simulink model "P2_SIL_Model_Diag"  (R2016a)
settings: Solver=ode2  StartTime=0.0  StopTime=Cycle_End  RelTol=1e-3
undefined symbols (not defined in the file): air, APP1_OOR, APP2_OOR, APP_Conversion_IN, APP_Mismatch, bms_inletair_temp, bms_maxchargecurrent, bms_maxdischargecurrent, BMS_Notfallkuehlung, BPP_Flt, cal, clt, ClutchEngag, CrankRequest, dcdc, eng, Engine, EngOverTemp, ENGTRQ_MSMCH_Degraded_CP, ENGTRQ_MSMCH_ErrCritical_CP, ENGTRQ_MSMCH_LimpHome_CP, EngTrqMismatch, env, ess, ESS, ESSOverTemp, fd, FFD, g, gb, Grade, IMG, KeyPos_Flt, KeyPosition, lib_APP_Conversion_IN, lib_ESS_plant_V1_2, lib_OBC_Manager, LossCAN, max_vehicle_rad_air_flow, MCUOverTemp, mot, MotDirMismatch, MotOverTemp, MotTrqMismatch, mph2kph, mph2ms, NeutralGear, obc, OBC_Manager, ParkGear, PRNDL_Flt, ReverseGear, RFD, rho, ShiftLeverPosition, sigbuilder_block, Speed, t_amb, time, tloop ... (+2)
libraries: simulink x104, EC2_libraries x12, Diagnostic x11, lib_CANerror_Detect x3, Utility x1
(part 1 of 11)
settings Model: SimulationMode=accelerator  Creator=Guilin  LastModifiedBy=Guilin
settings OptimizationCC: EfficientMapNaN2IntZero=off
settings HardwareCC: TargetBitPerPointer=64  TargetLongLongMode=on  TargetIntDivRoundTo=Zero  TargetEndianess=LittleEndian  TargetWordSize=64  TargetHWDeviceType=MATLAB Host  ProdEqTarget=off
settings CodeAppCC: MaxIdLength=128
settings GRTTargetCC: GeneratePreprocessorConditionals=Use local settings  CombineOutputUpdateFcns=off  GRTInterface=on

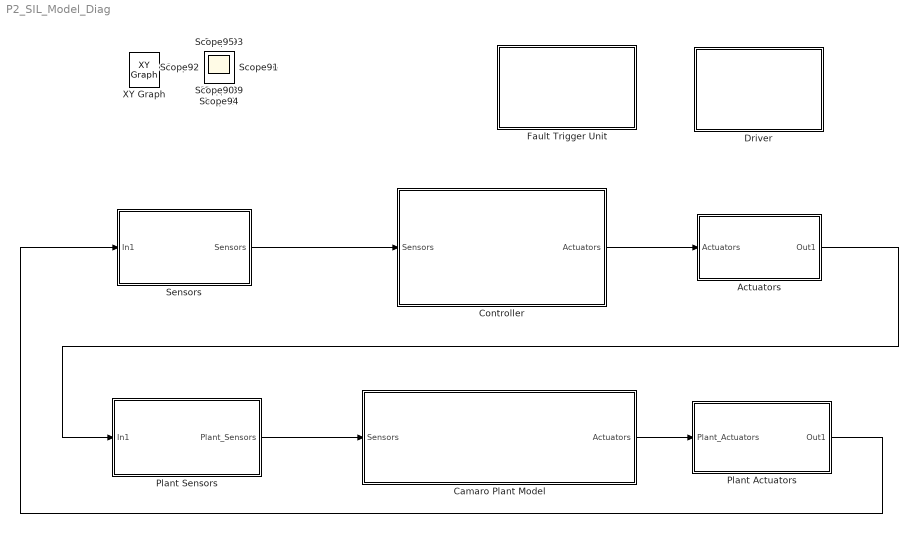
== system P2_SIL_Model_Diag ==
  Actuators : Subsystem
  Camaro Plant Model : Subsystem
      mask Display: image('Images\Vehicle.jpg')
  Controller : Subsystem
      mask Display: image('Images\HCU.jpg')
  Driver : Subsystem
      mask Display: image('Images\Driver.jpg')
  Fault Trigger Unit : Subsystem
  Plant Actuators : Subsystem
  Plant Sensors : Subsystem
  Sensors : Subsystem
  Scope{,1..95} (96 alike) : Scope
  XY Graph : simulink/Sinks/XY Graph  IOType=viewer  xmin=-1  xmax=1  ymin=-1  ymax=1  st=-1
  wires:
  Camaro Plant Model/1(Actuators) -> Plant Actuators/1(Plant_Actuators)
  Plant Sensors/1(Plant_Sensors) -> Camaro Plant Model/1(Sensors)
  Plant Actuators/1(Out1) -> Sensors/1(In1)
  Sensors/1(Sensors) -> Controller/1(Sensors)
  Controller/1(Actuators) -> Actuators/1(Actuators)
  Actuators/1(Out1) -> Plant Sensors/1(In1)

== system P2_SIL_Model_Diag/Actuators ==
  Actuators : Inport
  Analog : Subsystem
  Bus Creator : BusCreator  Inputs=3
  CAN : Subsystem
  Digital : Subsystem
  Ground : Ground
  Out1 : Outport
  wires:
  CAN/1(Out1) -> Bus Creator/1  "to_CAN"
  Analog/1(Out1) -> Bus Creator/2  "to_Analog"
  Digital/1(Out1) -> Bus Creator/3  "to_Digital"
  Actuators/1 -> Digital/1(In1), CAN/1(In1)
  Ground/1 -> Analog/1(In1)
  Bus Creator/1 -> Out1/1

== system P2_SIL_Model_Diag/Camaro Plant Model ==
  Sensors : Inport
  Add : Sum  Inputs=+++
      mask Display:
      | port_label('input',1,'+');
      | port_label('input',2,'+');
      | port_label('input',3,'+');
  Bus Creator : BusCreator  Inputs=2
  Bus Creator1 : BusCreator  Inputs=7
  Bus Selector : BusSelector  OutputSignals=Analog,CAN.to VEH_CAN,CAN.to EBCAN,CAN.to HV_CAN,Digital
  Chassis1 : Subsystem  AncestorBlock=Chassis/Chassis
      mask Display:
      | image('Images/Chassis.jpg');
      | color('red');
      | port_label('input',1,'ShaftIn');
      | port_label('output',1,'SpdOut');
  DC-DC Converter1 : Subsystem  AncestorBlock=DCDC/DC-DC Converter
      mask Display:
      | image('Images\DCDC.png')
      | color('red');
      | port_label('Input',1,'Volt')
      | port_label('Output',1,'Crr')
  Differential : Subsystem  AncestorBlock=Differential/Differential
      mask Display:
      | image('Images/Diff.jpg');
      | color('red');
      | port_label('input',1,'ShaftIn')
      | port_label('input',2,'SpdOut')
      | port_label('output',1,'ShaftOut')
      | port_label('output',2,'SpdIn')
  ESS : Subsystem  AncestorBlock=lib_ESS_plant_V1_2/ESS
      mask Display:
      | image('Images\ESS.jpg')
      | color('red');
      | port_label('Input',1,'Crr');
      | port_label('Output',1,'Volt');
  ICE Simple1 : Subsystem  AncestorBlock=Engine_simple/ICE Simple
      mask Display:
      | image(imread('EngineTopLevel.jpg'),'center')
      | color('red');
      | port_label('input',1,'SpdOut')
      | port_label('output',1,'ShaftOut')
  IMG : Subsystem  AncestorBlock=IMG/IMG
      mask Display:
      | image('Images\Motor.png')
      | color('red');
      | port_label('Input',1,'Volt');
      | port_label('Input',2,'ShaftIn');
      | port_label('Input',3,'SpdOut');
      | port_label('Output',1,'Crr');
      | port_label('Output',2,'ShaftOut');
      | port_label('Output',3,'SpdIn');
  On-Board Charger : Subsystem  AncestorBlock=OBC/On-Board Charger
      mask Display:
      | image('Images\OBC.jpg')
      | color('red');
      | port_label('Input',1,'Volt')
      | port_label('Output',1,'Crr')
  Scopes : Subsystem
      mask Display: image('Images\Scope.jpg')
  Transmission1 : Subsystem  AncestorBlock=Transmission/Transmission
      mask Display:
      | image('Images\Trans.png')
      | color('red');
      | port_label('Input',1,'ShaftIn')
      | port_label('Input',2,'SpdOut')
      | port_label('Output',1,'ShaftOut')
      | port_label('Output',2,'SpdIn')
  Wheels : Subsystem  AncestorBlock=Wheels/Wheels
      mask Display:
      | image('Images/Wheel.jpg');
      | color('red');
      | port_label('input',1,'ShaftIn');
      | port_label('input',2,'SpdOut');
      | port_label('output',1,'ShaftOut');
      | port_label('output',2,'SpdIn');
  Actuators : Outport
  tag scope: Analog=global, Digital=global, HCU_to_EBCAN=global, HCU_to_HV_CAN=global, HCU_to_VEH_CAN=global
  wires:
  Differential/1(fd_shaft_out) -> Wheels/1(whl_shaft_in)
  Wheels/1(whl_shaft_out) -> Chassis1/1(chas_shaft_in)
  Chassis1/1(chas_lin_spd_out) -> Wheels/2(whl_lin_spd_out)
  Differential/2(fd_spd_in) -> Transmission1/2(SpdOut)
  Transmission1/1(ShaftOut) -> Differential/1(fd_shaft_in)
  ESS/1(voltage) -> DC-DC Converter1/1(Volt), IMG/1(voltage), On-Board Charger/1(volt)
  DC-DC Converter1/1(Crr) -> Add/3
  On-Board Charger/1(crr) -> Add/2
  Add/1 -> ESS/1(current)
  Transmission1/2(SpdIn) -> IMG/3(IMG_SpdOut)
  IMG/2(IMG_ShaftOut) -> Transmission1/1(ShaftIn)
  IMG/1(current) -> Add/1
  Bus Creator/1 -> Actuators/1
  Sensors/1 -> Bus Selector/1
  Bus Selector/1 -> [Analog]  "<Analog>"
  Bus Selector/2 -> [HCU_to_VEH_CAN]  "<to VEH_CAN>"
  Bus Selector/3 -> [HCU_to_EBCAN]  "<to EBCAN>"
  Bus Selector/4 -> [HCU_to_HV_CAN]  "<to HV_CAN>"
  Bus Selector/5 -> [Digital]  "<Digital>"
  Wheels/2(whl_spd_in) -> Differential/2(fd_spd_out)
  ICE Simple1/1(eng_shaft_out) -> IMG/2(IMG_ShaftIn)
  IMG/3(IMG_SpdIn) -> ICE Simple1/1(eng_spd_out)
  [ECM_to_HCU] -> Bus Creator1/1
  [TCM_to_HCU] -> Bus Creator1/2
  [BCM_to_HCU] -> Bus Creator1/3
  [BMS_to_HCU] -> Bus Creator1/4
  [MCU_to_HCU] -> Bus Creator1/5
  [APM_to_HCU] -> Bus Creator1/6
  [OBC_to_HCU] -> Bus Creator1/7
  Bus Creator1/1 -> Bus Creator/1  "CAN_to_Actuators"
  [Driver_Request] -> Bus Creator/2  "Driver_Signals"

== system P2_SIL_Model_Diag/Controller ==
  Sensors : Inport
  HSC : Subsystem
  Actuators : Outport
  wires:
  Sensors/1 -> HSC/1(Sensors)
  HSC/1(Actuators) -> Actuators/1

== system P2_SIL_Model_Diag/Driver ==
  Bus Creator : BusCreator  Inputs=6
  Constant : Constant  Commented=on  Value=0
  Driver Control : Subsystem
  Manual Control : Subsystem  Commented=on
  Multiport Switch1 : MultiPortSwitch  Commented=on  DataPortOrder=Zero-based contiguous  Inputs=2
  tag scope: Driver_Request=global
  wires:
  Driver Control/1(Key Position) -> Bus Creator/1  "KeyPos"
  Driver Control/2(APP[%]) -> Bus Creator/2  "drv_APP_req_[%]"
  Driver Control/3(BPP[%]) -> Bus Creator/3  "drv_BPP_req_[%]"
  Driver Control/4(Shift Lever Position) -> Bus Creator/4  "ShiftLvrPos"
  Driver Control/5(EVSE_Pluggin) -> Bus Creator/5  "EVSE_Plugged"
  Constant/1 -> Multiport Switch1/1
  Manual Control/1(Out1) -> Multiport Switch1/3
  Bus Creator/1 -> [Driver_Request]
  Driver Control/6(Veh_Spd) -> Bus Creator/6  "Veh_Spd"

== system P2_SIL_Model_Diag/Fault Trigger Unit ==
  Clock3 : Clock
  Component Diagnostics setting : Subsystem
  Driver Interface Diagnostics setting : Subsystem
  wires:
  Clock3/1 -> Component Diagnostics setting/1(time), Driver Interface Diagnostics setting/1(time)

== system P2_SIL_Model_Diag/Plant Actuators ==
  Plant_Actuators : Inport
  Analog : Subsystem
  Bus Creator : BusCreator  Inputs=3
  Bus Selector : BusSelector  OutputSignals=CAN_to_Actuators,Driver_Signals
  CAN : Subsystem
  Digital : Subsystem  Commented=on
  Out1 : Outport
  wires:
  Bus Creator/1 -> Out1/1  "to_HCU_Sensors"
  Bus Selector/2 -> Analog/1(In1), Digital/1(In1)  "<Driver_Signals>"
  Bus Selector/1 -> CAN/1(In1)  "<CAN_to_Actuators>"
  Plant_Actuators/1 -> Bus Selector/1
  Analog/1(Out1) -> Bus Creator/2  "Analog_to_HCU_Sensors"
  CAN/1(Out1) -> Bus Creator/1  "CAN_to_HCU_Sensors"

== system P2_SIL_Model_Diag/Plant Sensors ==
  In1 : Inport
  Analog : Subsystem
  Bus Creator : BusCreator  Inputs=3
  Bus Selector : BusSelector  OutputSignals=to_CAN,to_Analog,to_Digital
  CAN : Subsystem
  Digital : Subsystem
  Plant_Sensors : Outport
  wires:
  Bus Creator/1 -> Plant_Sensors/1
  Digital/1(Out1) -> Bus Creator/3  "Digital"
  Analog/1(Out1) -> Bus Creator/2  "Analog"
  CAN/1(Out1) -> Bus Creator/1  "CAN"
  In1/1 -> Bus Selector/1
  Bus Selector/1 -> CAN/1(In1)  "<to_CAN>"
  Bus Selector/2 -> Analog/1(In1)  "<to_Analog>"
  Bus Selector/3 -> Digital/1(In1)  "<to_Digital>"

== system P2_SIL_Model_Diag/Sensors ==
  In1 : Inport
  Analog : Subsystem
  Bus Creator : BusCreator  Inputs=3
  Bus Selector : BusSelector  OutputSignals=CAN_to_HCU_Sensors,Analog_to_HCU_Sensors
  CAN : Subsystem
  Digital : Subsystem  Commented=on
  Memory : Memory
  Sensors : Outport
  wires:
  Analog/1(Out1) -> Bus Creator/2  "from_Analog"
  CAN/1(Out1) -> Bus Creator/1  "from_CAN"
  In1/1 -> Bus Selector/1
  Bus Selector/1 -> CAN/1(In1)  "<CAN_to_HCU_Sensors>"
  Bus Selector/2 -> Analog/1(In1)  "<Analog_to_HCU_Sensors>"
  ? -> Digital/1(In1)  "<Digital_to_HCU_Sensors>"
  Bus Creator/1 -> Memory/1
  Memory/1 -> Sensors/1

== system P2_SIL_Model_Diag/Actuators/Analog ==
  In1 : Inport
  Out1 : Outport
  wires:
  In1/1 -> Out1/1

== system P2_SIL_Model_Diag/Actuators/CAN ==
  In1 : Inport
  Bus Creator : BusCreator  Inputs=3
  EBCAN : Subsystem
  HV_CAN : Subsystem
  VEH_CAN : Subsystem
  Out1 : Outport
  wires:
  VEH_CAN/1(Out1) -> Bus Creator/1  "to_VEH_CAN"
  EBCAN/1(Out1) -> Bus Creator/2  "to_EBCAN"
  HV_CAN/1(Out1) -> Bus Creator/3  "to_HV_CAN"
  Bus Creator/1 -> Out1/1  "to_CAN"
  In1/1 -> HV_CAN/1(In1), EBCAN/1(In1), VEH_CAN/1(In1)

== system P2_SIL_Model_Diag/Actuators/Digital ==
  In1 : Inport
  Bus Selector : BusSelector  OutputSignals=BMS_Digital
  Out1 : Outport
  wires:
  In1/1 -> Bus Selector/1
  Bus Selector/1 -> Out1/1  "<BMS_Digital>"

== system P2_SIL_Model_Diag/Camaro Plant Model/Chassis1 ==
  note: Total opposing
      | force (N)
  chas_shaft_in : Inport
  >1 : Saturate  UpperLimit=inf  LowerLimit=0
  Bus Selector : BusSelector  OutputSignals=veh_grade_force_simu,drag force
  Bus Selector1 : BusSelector  OutputSignals=whl_force_out_simu,whl_mass_out_simu
  Clock : Clock
  Driver Interface : Subsystem
  Grade : Lookup  InputValues=time  Table=Grade
  Soft BCM : Subsystem
      mask Display: image('SoftECU.jpg')
  Sum2 : Sum  Inputs=|++  SaturateOnIntegerOverflow=on  InputSameDT=on  OutDataTypeStr=Inherit: Same as first input
  Sum3 : Sum  Inputs=-+  SaturateOnIntegerOverflow=on  InputSameDT=on  OutDataTypeStr=Inherit: Same as first input
  To Workspace1 : ToWorkspace  VariableName=distance_miles_hist  SampleTime=-1
      settings: Decimation=WORKSPACE_DECIMATION
  To Workspace2 : ToWorkspace  VariableName=veh_dist_meter_hist  SampleTime=-1
      settings: Decimation=WORKSPACE_DECIMATION
  To Workspace3 : ToWorkspace  VariableName=veh_spd_mps_hist  SampleTime=-1
      settings: Decimation=WORKSPACE_DECIMATION
  To Workspace7 : ToWorkspace  VariableName=veh_spd_mph_hist  SampleTime=-1
      settings: Decimation=WORKSPACE_DECIMATION
  Velocity1 : Integrator  LimitOutput=on  LowerSaturationLimit=0
  Velocity2 : Integrator  LimitOutput=on  LowerSaturationLimit=0
  m to miles : Gain  Gain=0.00062
  m/s to kph : Gain  Gain=3.6
  ms to mph : Gain  Gain=1/mph2ms
  non-zero division1 : Subsystem
      mask Display: disp('divider \n I1/I2')
  vehicle losses : Subsystem
  vehicle total mass : Constant  Value=veh.init.mass
  chas_lin_spd_out : Outport
  tag scope: BCM_to_HCU=global, chas_plant_force_in=global, chas_plant_force_loss=global, chas_plant_grade=global, chas_plant_lin_accel=global, chas_plant_lin_spd_out=global, chas_plant_mass=global, chas_plant_mass_static=global, veh_dist_miles=global
  wires:
  Grade/1 -> vehicle losses/2(Road grade), [chas_plant_grade]
  Bus Selector/2 -> [chas_plant_force_loss]  "<drag force>"
  Bus Selector/1 -> [chas_plant_force_grade]  "<veh_grade_force_simu>"
  vehicle total mass/1 -> Sum2/1, [chas_plant_mass_static]
  Velocity1/1 -> vehicle losses/1(veh spd simu), m/s to kph/1, Velocity2/1, To Workspace3/1, ms to mph/1, chas_lin_spd_out/1
  non-zero division1/1(Out1) -> Velocity1/1, [chas_plant_lin_accel]
  Sum3/1 -> non-zero division1/1(In1)
  Sum2/1 -> non-zero division1/2(In2), [chas_plant_mass]
  >1/1 -> Sum2/2
  Bus Selector1/2 -> >1/1  "<whl_mass_out_simu>"
  Bus Selector1/1 -> Sum3/2, [chas_plant_force_in]  "<whl_force_out_simu>"
  chas_shaft_in/1 -> Bus Selector1/1
  vehicle losses/1(info) -> Bus Selector/1
  vehicle losses/2(veh_force_loss_simu) -> Sum3/1
  Soft BCM/1(Out1) -> [BCM_to_HCU]
  m/s to kph/1 -> [chas_plant_lin_spd_out]
  ms to mph/1 -> To Workspace7/1
  Clock/1 -> Grade/1
  Velocity2/1 -> To Workspace2/1, m to miles/1
  m to miles/1 -> [veh_dist_miles], To Workspace1/1

== system P2_SIL_Model_Diag/Camaro Plant Model/DC-DC Converter1 ==
  Volt : Inport
  Eff : Gain  Gain=1/dcdc.init.eff
  Electrical Accessory Load : Constant  Value=dcdc.init.constant_pwr
  Subsystem2 : Subsystem
      mask Display: disp('divider')
  Crr : Outport
  wires:
  Eff/1 -> Subsystem2/1(In1)
  Subsystem2/1(Out1) -> Crr/1
  Electrical Accessory Load/1 -> Eff/1
  Volt/1 -> Subsystem2/2(In2)

== system P2_SIL_Model_Diag/Camaro Plant Model/Differential ==
  fd_shaft_in : Inport
  fd_spd_out : Inport  Port=2
  Bus Creator : BusCreator  Inputs=2
  Bus Selector : BusSelector  OutputSignals=gb_trq_out,gb_inertia_out
  Inertia calculation : Subsystem
  Speed calculation : Subsystem
  Torque calculation : Subsystem
  fd_shaft_out : Outport
  fd_spd_in : Outport  Port=2
  wires:
  Torque calculation/1(trq out) -> Bus Creator/1  "fd_trq_out_simu"
  fd_spd_out/1 -> Speed calculation/1(spd out)
  Speed calculation/1(spd in) -> Torque calculation/1(spd in), fd_spd_in/1
  Inertia calculation/1(inertia out) -> Bus Creator/2  "fd_inertia_out_simu"
  Bus Selector/1 -> Torque calculation/2(trq in)  "<gb_trq_out>"
  Bus Selector/2 -> Inertia calculation/1(inertia in)  "<gb_inertia_out>"
  fd_shaft_in/1 -> Bus Selector/1
  Bus Creator/1 -> fd_shaft_out/1

== system P2_SIL_Model_Diag/Camaro Plant Model/ESS ==
  note: BMS_to_Actuators
  current : Inport
  ESS : Subsystem
      mask Display:
      | image('Images\ESS.jpg')
      | color('red');
      | port_label('Input',2,'Crr');
      | port_label('Output',2,'Volt');
  Inputs : Subsystem  AncestorBlock=lib_DCDC/DC-DC Converter/Inputs
  Outputs : Subsystem
  Soft BMS : Subsystem  RequirementInfo={} %GIDa_a1686922_eaef_470c_99b9_57900de5863a
      mask Display: image('softECU.jpg')
  voltage : Outport
  wires:
  current/1 -> ESS/2("Crr ")
  Soft BMS/2(Output2) -> ESS/1("In ")
  ESS/1(out) -> Soft BMS/2(Input2)  "Sensors_to_BMS"
  ESS/2(Voltage) -> voltage/1
  Soft BMS/1(CAN) -> Outputs/1(Outputs)
  Inputs/1(Inputs) -> Soft BMS/1(Input1)

== system P2_SIL_Model_Diag/Camaro Plant Model/ICE Simple1 ==
  eng_spd_out : Inport
  Engine Plant Modified : Subsystem
      mask Display:
      | image(imread('EngineTopLevel.jpg'),'center')
      | color('red');
      | port_label('input',2,'SpdOut')
      | port_label('output',2,'ShaftOut')
  Inputs : Subsystem
  Soft ECM : Subsystem
      mask Display: image('SoftECU.jpg')
  eng_shaft_out : Outport
  tag scope: ECM_to_HCU=global
  wires:
  Engine Plant Modified/2(eng_shaft_out) -> eng_shaft_out/1
  eng_spd_out/1 -> Engine Plant Modified/2(eng_spd_out)
  Soft ECM/2(Out1) -> Engine Plant Modified/1("In ")  "ECM_to_Actuators"
  Inputs/1(Inputs) -> Soft ECM/1(In)
  Soft ECM/1(Out) -> [ECM_to_HCU]
  Engine Plant Modified/1(Out) -> Soft ECM/2(In1)

== system P2_SIL_Model_Diag/Camaro Plant Model/IMG ==
  voltage : Inport
  IMG_ShaftIn : Inport  Port=2
  IMG_SpdOut : Inport  Port=3
  IMG Plant : Subsystem
      mask Display:
      | image('Images\Motor.png')
      | color('red');
      | port_label('Input',2,'Volt');
      | port_label('Input',3,'ShaftIn');
      | port_label('Input',4,'SpdOut');
      | port_label('Output',2,'Crr');
      | port_label('Output',3,'ShaftOut');
      | port_label('Output',4,'SpdIn');
  Soft MCU : Subsystem
      mask Display: image('softECU.jpg')
  current : Outport
  IMG_ShaftOut : Outport  Port=2
  IMG_SpdIn : Outport  Port=3
  tag scope: MCU_to_HCU=global
  wires:
  IMG Plant/1(Out1) -> Soft MCU/2(In1)  "Sensors_to_MCU"
  Soft MCU/2(Out1) -> IMG Plant/1("In1 ")  "MCU_to_Actuators"
  Soft MCU/1(Out) -> [MCU_to_HCU]
  [HCU_to_HV_CAN] -> Soft MCU/1(In)
  IMG_SpdOut/1 -> IMG Plant/4(SpdOut)
  IMG Plant/4(SpdIn) -> IMG_SpdIn/1
  IMG Plant/2(current) -> current/1
  voltage/1 -> IMG Plant/2(voltage)
  IMG Plant/3(MotShaftOut) -> IMG_ShaftOut/1
  IMG_ShaftIn/1 -> IMG Plant/3(MotShaftIn)

== system P2_SIL_Model_Diag/Camaro Plant Model/On-Board Charger ==
  volt : Inport
  HCU to OBC : Subsystem
  OBC to HCU : Subsystem
  On Board Charger : Subsystem
      mask Display:
      | image('Images\OBC.jpg')
      | color('red');
      | port_label('Input',1,'Volt')
      | port_label('Output',1,'Crr')
  Soft_OBC : Subsystem
      mask Display: image('softECU.jpg')
  crr : Outport
  wires:
  volt/1 -> On Board Charger/2(volt)
  On Board Charger/2(crr) -> crr/1
  HCU to OBC/1(Inputs) -> Soft_OBC/1(Inputs)
  Soft_OBC/1(Outputs) -> OBC to HCU/1(Outputs)
  On Board Charger/1(Out1) -> Soft_OBC/2(Inputs1)  "Sensors_to_OBC"
  Soft_OBC/2(Outputs1) -> On Board Charger/1("In1 ")  "OBC_to_Actuators"

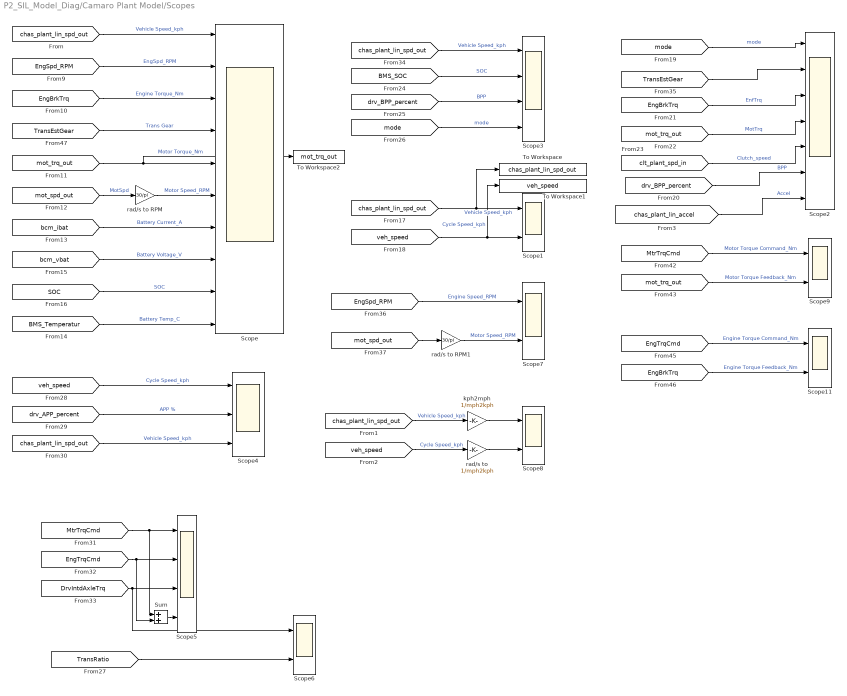
== system P2_SIL_Model_Diag/Camaro Plant Model/Scopes ==
  Scope : Scope  NumInputPorts=10
  Scope{1,6..9,11} (6 alike) : Scope  NumInputPorts=2
  Scope2 : Scope  NumInputPorts=7
  Scope3 : Scope  NumInputPorts=4
  Scope4 : Scope  NumInputPorts=3
  Scope5 : Scope  NumInputPorts=4
  Sum : Sum
  To Workspace : ToWorkspace  VariableName=chas_plant_lin_spd_out  SaveFormat=Timeseries  SampleTime=-1
  To Workspace1 : ToWorkspace  VariableName=veh_speed  SaveFormat=Timeseries  SampleTime=-1
  To Workspace2 : ToWorkspace  VariableName=mot_trq_out  SaveFormat=Timeseries  SampleTime=-1
  kph2mph : Gain  Gain=1/mph2kph
  "rad/s to " : Gain  Gain=1/mph2kph
  rad/s to RPM : Gain  Gain=30/pi
  rad/s to RPM1 : Gain  Gain=30/pi
  wires:
  [chas_plant_lin_spd_out] -> Scope/1  "Vehicle Speed_kph"
  [EngSpd_RPM] -> Scope/2  "EngSpd_RPM"
  [EngBrkTrq] -> Scope/3  "Engine Torque_Nm"
  [mot_spd_out] -> rad/s to RPM/1  "MotSpd"
  [BMS_Temperatur] -> Scope/10  "Battery Temp_C"
  rad/s to RPM/1 -> Scope/6  "Motor Speed_RPM"
  [mot_trq_out] -> To Workspace2/1, Scope/5  "Motor Torque_Nm"
  [bcm_vbat] -> Scope/8  "Battery Voltage_V"
  [SOC] -> Scope/9  "SOC"
  [TransEstGear] -> Scope/4  "Trans Gear"
  [bcm_ibat] -> Scope/7  "Battery Current_A"
  [chas_plant_lin_spd_out] -> Scope3/1  "Vehicle Speed_kph"
  [BMS_SOC] -> Scope3/2  "SOC"
  [drv_BPP_percent] -> Scope3/3  "BPP"
  [mode] -> Scope3/4  "mode"
  [chas_plant_lin_spd_out] -> To Workspace/1, Scope1/1  "Vehicle Speed_kph"
  [veh_speed] -> To Workspace1/1, Scope1/2  "Cycle Speed_kph"
  [mode] -> Scope2/1  "mode"
  [EngBrkTrq] -> Scope2/3  "EnfTrq"
  [mot_trq_out] -> Scope2/4  "MotTrq"
  [clt_plant_spd_in] -> Scope2/5  "Clutch_speed"
  [EngSpd_RPM] -> Scope7/1  "Engine Speed_RPM"
  [mot_spd_out] -> rad/s to RPM1/1
  rad/s to RPM1/1 -> Scope7/2  "Motor Speed_RPM"
  [veh_speed] -> Scope4/1  "Cycle Speed_kph"
  [drv_APP_percent] -> Scope4/2  "APP %"
  [chas_plant_lin_spd_out] -> Scope4/3  "Vehicle Speed_kph"
  [MtrTrqCmd] -> Sum/1, Scope5/1
  [EngTrqCmd] -> Sum/2, Scope5/2
  [DrvIntdAxleTrq] -> Scope6/1, Scope5/3
  Sum/1 -> Scope5/4
  [TransRatio] -> Scope6/2
  [MtrTrqCmd] -> Scope9/1  "Motor Torque Command_Nm"
  [mot_trq_out] -> Scope9/2  "Motor Torque Feedback_Nm"
  [EngTrqCmd] -> Scope11/1  "Engine Torque Command_Nm"
  [EngBrkTrq] -> Scope11/2  "Engine Torque Feedback_Nm"
  [chas_plant_lin_spd_out] -> kph2mph/1  "Vehicle Speed_kph"
  [veh_speed] -> "rad/s to "/1  "Cycle Speed_kph"
  kph2mph/1 -> Scope8/1
  "rad/s to "/1 -> Scope8/2
  [TransEstGear] -> Scope2/2
  [drv_BPP_percent] -> Scope2/6  "BPP"
  [chas_plant_lin_accel] -> Scope2/7  "Accel"

== system P2_SIL_Model_Diag/Camaro Plant Model/Transmission1 ==
  ShaftIn : Inport
  SpdOut : Inport  Port=2
  Inputs : Subsystem  AncestorBlock=lib_DCDC/DC-DC Converter/Inputs
  Outputs : Subsystem  AncestorBlock=lib_DCDC/DC-DC Converter/Outputs
  Soft TCM : Subsystem
      mask Display: image('softECU.jpg')
  Transmission Plant : Subsystem
      mask Display:
      | image('Images\Trans.png')
      | color('red');
      | port_label('Input',2,'ShaftIn')
      | port_label('Input',3,'SpdOut')
      | port_label('Output',2,'ShaftOut')
      | port_label('Output',3,'SpdIn')
  ShaftOut : Outport
  SpdIn : Outport  Port=2
  wires:
  Transmission Plant/3(TorqConvSpdIn) -> SpdIn/1
  Transmission Plant/2(GearboxShaftOut) -> ShaftOut/1
  SpdOut/1 -> Transmission Plant/3(GearboxSpdOut)
  ShaftIn/1 -> Transmission Plant/2(TorqConvShaftIn)
  Soft TCM/1(Out) -> Outputs/1(Outputs)
  Inputs/1(Inputs) -> Soft TCM/1(In)
  Transmission Plant/1(Out1) -> Soft TCM/2(In1)  "Sensors_to_TCM"
  Soft TCM/2(Out1) -> Transmission Plant/1("In1 ")  "TCM_to_Actuators"

== system P2_SIL_Model_Diag/Camaro Plant Model/Wheels ==
  whl_shaft_in : Inport
  whl_lin_spd_out : Inport  Port=2
  "1\\radius " : Gain  Gain=1/whl.plant.init.radius  SaturateOnIntegerOverflow=on  OutDataTypeStr=Inherit: Same as input  ParamDataTypeStr=Inherit: Same as input
  Bus Creator : BusCreator  Inputs=2
  Bus Selector : BusSelector  OutputSignals=drv_BPP_req_[%]
  Bus Selector1 : BusSelector  OutputSignals=fd_trq_out_simu,fd_inertia_out_simu
  Clock : Clock
  Force calculation : Subsystem
  Grade : Lookup  InputValues=time  Table=Grade
  Mass calculation : Subsystem
  Speed calculation : Subsystem
  whl_shaft_out : Outport
  whl_spd_in : Outport  Port=2
  wires:
  Bus Selector/1 -> Force calculation/2(BPP[%])  "<drv_BPP_req_[%]>"
  [Driver_Request] -> Bus Selector/1
  "1\\radius "/1 -> Speed calculation/1(chas_spd)
  Force calculation/1(force) -> Bus Creator/1  "whl_force_out_simu"
  Speed calculation/1(spd in) -> Force calculation/1(spd in), whl_spd_in/1
  Mass calculation/1(Mass) -> Bus Creator/2  "whl_mass_out_simu"
  Bus Selector1/1 -> Force calculation/5(trq_in)  "<fd_trq_out_simu>"
  Bus Selector1/2 -> Mass calculation/1(inertia in)  "<fd_inertia_out_simu>"
  whl_lin_spd_out/1 -> "1\\radius "/1, Force calculation/3(whl_spd)
  whl_shaft_in/1 -> Bus Selector1/1
  Bus Creator/1 -> whl_shaft_out/1
  Grade/1 -> Force calculation/4(grade)
  Clock/1 -> Grade/1

== system P2_SIL_Model_Diag/Controller/HSC ==
  Sensors : Inport
  Camaro Fault Detection : Subsystem  AncestorBlock=Diagnostic/Camaro Diagnostic
  Driver_Requests : Subsystem  RequirementInfo="{'other' 'HCU_Requirements.xlsx' '@Simulink_requirement_item_5' 'true' 'Determines the  driver''s intention i.e. status of the vehicle start, HCU on/off status and the Driver Intend Axle Torque from the sensor inputs.' '' } %GIDa_43b9b296_ab65_412c_9ca4_dcb3f85d1554"
  Ground : Ground
  Powertrain Manager : Subsystem
  Actuators : Outport
  wires:
  Sensors/1 -> Driver_Requests/1(Sensors), Camaro Fault Detection/1(Sensors), Powertrain Manager/1(Sensors)
  Powertrain Manager/1(Out1) -> Actuators/1
  Ground/1 -> Driver_Requests/2(Diagnostics)
  Driver_Requests/1(DriverRequests) -> Powertrain Manager/2(Driver Request)
  Camaro Fault Detection/1(Out2) -> Powertrain Manager/3(Fault Detection)

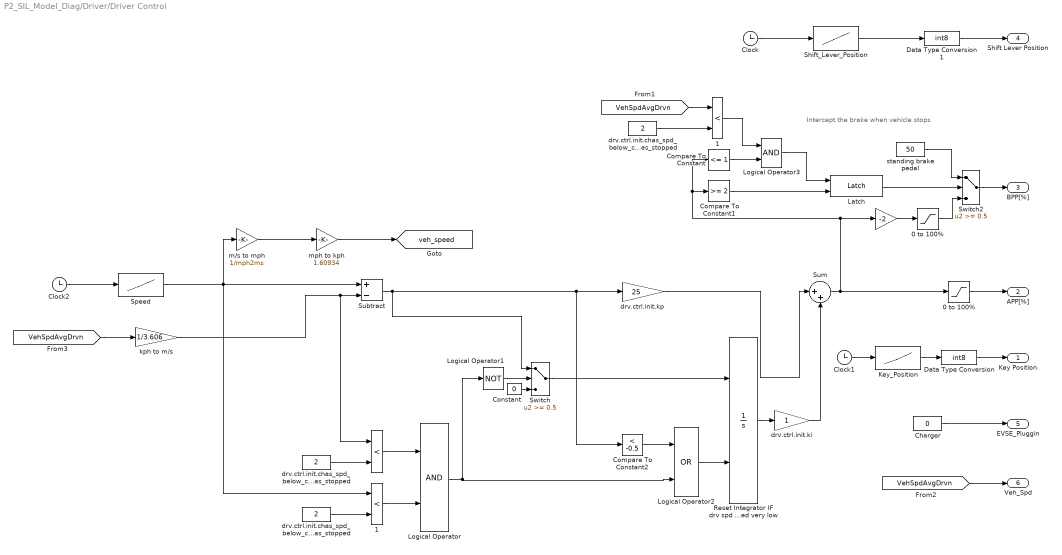
== system P2_SIL_Model_Diag/Driver/Driver Control ==
  note: Intercept the brake when vehicle stops
  " " : Gain  Gain=-2
  "    " : RelationalOperator  Operator=<  InputSameDT=on
  "    1" : RelationalOperator  Operator=<  InputSameDT=on
  "  1" : RelationalOperator  Operator=<  InputSameDT=on
  0 to 100% : Saturate  UpperLimit=100  LowerLimit=0
  "0 to 100% " : Saturate  UpperLimit=100  LowerLimit=0
  Charger : Constant  Value=0
  Clock : Clock
  Clock1 : Clock
  Clock2 : Clock
  Compare To Constant : simulink/Logic and Bit Operations/Compare To Constant  relop=<=  const=1  OutDataTypeStr=boolean
  Compare To Constant1 : simulink/Logic and Bit Operations/Compare To Constant  relop=>=  const=2  OutDataTypeStr=boolean
  Compare To Constant2 : simulink/Logic and Bit Operations/Compare To Constant  relop=<  const=-0.5  OutDataTypeStr=boolean
  Constant : Constant  Value=0
  Data Type Conversion : DataTypeConversion  OutDataTypeStr=int8
  Data Type Conversion1 : DataTypeConversion  OutDataTypeStr=int8
  Key_Position : Lookup  InputValues=time  Table=KeyPosition
  Latch : Utility/Latch
  Logical Operator : Logic  AllPortsSameDT=off  OutDataTypeStr=boolean
  Logical Operator1 : Logic  Operator=NOT  AllPortsSameDT=off  OutDataTypeStr=boolean
  Logical Operator2 : Logic  Operator=OR  AllPortsSameDT=off  OutDataTypeStr=boolean
  Logical Operator3 : Logic  AllPortsSameDT=off  OutDataTypeStr=boolean
  Reset Integrator IF drv spd dmd very low AND AND current vehicle speed very low : Integrator  ExternalReset=either
  Shift_Lever_Position : Lookup  InputValues=time  Table=ShiftLeverPosition
  Speed : Lookup  InputValues=time  Table=Speed
  Subtract : Sum  Inputs=+-
  Sum : Sum  Inputs=|++  SaturateOnIntegerOverflow=on  InputSameDT=on  OutDataTypeStr=Inherit: Same as first input
  Switch : Switch  Threshold=0.5
  Switch2 : Switch  Threshold=0.5
  "drv.ctrl.init.chas_spd_below_chas_stopped " : Constant  Value=2
  "drv.ctrl.init.chas_spd_below_chas_stopped " : Constant  Value=2
  "drv.ctrl.init.chas_spd_below_chas_stopped " : Constant  Value=2
  drv.ctrl.init.ki : Gain  SaturateOnIntegerOverflow=on  OutDataTypeStr=Inherit: Same as input  ParamDataTypeStr=Inherit: Same as input
  drv.ctrl.init.kp : Gain  Gain=25  SaturateOnIntegerOverflow=on  OutDataTypeStr=Inherit: Same as input  ParamDataTypeStr=Inherit: Same as input
  kph to m/s : Gain  Gain=1/3.606  SaturateOnIntegerOverflow=on  OutDataTypeStr=Inherit: Same as input  ParamDataTypeStr=Inherit: Same as input
  m/s to mph : Gain  Gain=1/mph2ms
  mph to kph : Gain  Gain=1.60934
  standing brake pedal : Constant  Value=50
  Key Position : Outport
  APP[%] : Outport  Port=2
  BPP[%] : Outport  Port=3
  Shift Lever Position : Outport  Port=4
  EVSE_Pluggin : Outport  Port=5
  Veh_Spd : Outport  Port=6
  tag scope: veh_speed=global
  wires:
  drv.ctrl.init.kp/1 -> Sum/1
  "    "/1 -> Logical Operator/1
  Speed/1 -> Subtract/1, m/s to mph/1, "  1"/1
  Constant/1 -> Switch/3
  Reset Integrator IF drv spd dmd very low AND AND current vehicle speed very low/1 -> drv.ctrl.init.ki/1
  kph to m/s/1 -> Subtract/2, "    "/1
  Logical Operator1/1 -> Switch/2
  "drv.ctrl.init.chas_spd_below_chas_stopped "/1 -> "    "/2
  Switch/1 -> Reset Integrator IF drv spd dmd very low AND AND current vehicle speed very low/1
  Logical Operator2/1 -> Reset Integrator IF drv spd dmd very low AND AND current vehicle speed very low/2
  "drv.ctrl.init.chas_spd_below_chas_stopped "/1 -> "  1"/2
  drv.ctrl.init.ki/1 -> Sum/2
  "  1"/1 -> Logical Operator/2
  Logical Operator/1 -> Logical Operator2/2, Logical Operator1/1
  "0 to 100% "/1 -> Switch2/3
  " "/1 -> "0 to 100% "/1
  [VehSpdAvgDrvn] -> kph to m/s/1
  standing brake pedal/1 -> Switch2/1
  Switch2/1 -> BPP[%]/1
  [VehSpdAvgDrvn] -> "    1"/1
  "drv.ctrl.init.chas_spd_below_chas_stopped "/1 -> "    1"/2
  "    1"/1 -> Logical Operator3/1
  Sum/1 -> Compare To Constant1/1, Compare To Constant/1, " "/1, 0 to 100%/1
  Logical Operator3/1 -> Latch/1
  Compare To Constant/1 -> Logical Operator3/2
  Compare To Constant1/1 -> Latch/2
  Latch/1 -> Switch2/2
  Shift_Lever_Position/1 -> Data Type Conversion1/1
  Data Type Conversion/1 -> Key Position/1
  Data Type Conversion1/1 -> Shift Lever Position/1
  Charger/1 -> EVSE_Pluggin/1
  Subtract/1 -> Compare To Constant2/1, drv.ctrl.init.kp/1, Switch/1
  Compare To Constant2/1 -> Logical Operator2/1
  Clock/1 -> Shift_Lever_Position/1
  Clock1/1 -> Key_Position/1
  Key_Position/1 -> Data Type Conversion/1
  Clock2/1 -> Speed/1
  m/s to mph/1 -> mph to kph/1
  mph to kph/1 -> [veh_speed]
  0 to 100%/1 -> APP[%]/1
  [VehSpdAvgDrvn] -> Veh_Spd/1

== system P2_SIL_Model_Diag/Driver/Manual Control ==
  note: Manipulate these values
      | to drive vehicle
  APP[%] : Constant
  BPP[%] : Constant  Value=-1
  Bus Creator1 : BusCreator  Inputs=5
  KeyPosition : Constant  Value=3
  PRNDL : Constant  Value=4
  ReferenceVel1 : Constant  Value=0
  Saturation : Saturate  UpperLimit=100  LowerLimit=0
  Saturation1 : Saturate  UpperLimit=0  LowerLimit=-100
  Saturation2 : Saturate  UpperLimit=3  LowerLimit=0
  Saturation3 : Saturate  UpperLimit=4  LowerLimit=0
  Slider Gain : simulink/Math Operations/Slider Gain  low=0  gain=0  high=100
  Slider Gain1 : simulink/Math Operations/Slider Gain  low=0  gain=0  high=100
  Out1 : Outport
  wires:
  Saturation2/1 -> Bus Creator1/3  "Key_Pos_[0_3]"
  Saturation1/1 -> Bus Creator1/2  "BPP(%)"
  Saturation/1 -> Bus Creator1/1  "APP (%)"
  KeyPosition/1 -> Saturation2/1
  Bus Creator1/1 -> Out1/1  "DriverOut"
  BPP[%]/1 -> Slider Gain1/1
  APP[%]/1 -> Slider Gain/1
  ReferenceVel1/1 -> Bus Creator1/5  "refVel [m/s]"
  PRNDL/1 -> Saturation3/1
  Saturation3/1 -> Bus Creator1/4  "PRNDL"
  Slider Gain/1 -> Saturation/1
  Slider Gain1/1 -> Saturation1/1

== system P2_SIL_Model_Diag/Fault Trigger Unit/Component Diagnostics setting ==
  time : Inport
  ClutchEngag : Lookup  Commented=on  InputValues=time  Table=ClutchEngag  LookUpMeth=Interpolation-Use End Values  OutDataTypeStr=int8
  ESSOverTemp : Lookup  Commented=on  InputValues=time  Table=ESSOverTemp  LookUpMeth=Interpolation-Use End Values  OutDataTypeStr=int8
  EngOverTemp : Lookup  Commented=on  InputValues=time  Table=EngOverTemp  LookUpMeth=Interpolation-Use End Values  OutDataTypeStr=int8
  EngTrqMismatch : Lookup  Commented=on  InputValues=time  Table=EngTrqMismatch  LookUpMeth=Interpolation-Use End Values  OutDataTypeStr=int8
  Goto1 : Goto  Commented=on  GotoTag=MotTrqMismatch  TagVisibility=global
  Goto2 : Goto  Commented=on  GotoTag=LossCAN_ON  TagVisibility=global
  Goto3 : Goto  Commented=on  GotoTag=EngTrqMismatch  TagVisibility=global
  Goto4 : Goto  Commented=on  GotoTag=MotOverTemp  TagVisibility=global
  Goto5 : Goto  Commented=on  GotoTag=MCUOverTemp  TagVisibility=global
  Goto6 : Goto  Commented=on  GotoTag=MotDirMismatch  TagVisibility=global
  Goto7 : Goto  Commented=on  GotoTag=EngOverTemp  TagVisibility=global
  Goto8 : Goto  Commented=on  GotoTag=ESSOverTemp  TagVisibility=global
  Goto9 : Goto  Commented=on  GotoTag=ClutchEngagFlt  TagVisibility=global
  LossCAN : Lookup  Commented=on  InputValues=time  Table=LossCAN  LookUpMeth=Interpolation-Use End Values  OutDataTypeStr=int8
  MCUOverTemp : Lookup  Commented=on  InputValues=time  Table=MCUOverTemp  LookUpMeth=Interpolation-Use End Values  OutDataTypeStr=int8
  Mismch type : Subsystem  Commented=on
  Mismch type1 : Subsystem  Commented=on
  MotDirMismatch : Lookup  Commented=on  InputValues=time  Table=MotDirMismatch  LookUpMeth=Interpolation-Use End Values  OutDataTypeStr=int8
  MotOverTemp : Lookup  Commented=on  InputValues=time  Table=MotOverTemp  LookUpMeth=Interpolation-Use End Values  OutDataTypeStr=int8
  MotTrqMismatch : Lookup  Commented=on  InputValues=time  Table=MotTrqMismatch  LookUpMeth=Interpolation-Use End Values  OutDataTypeStr=int8
  Override  ClutchEngag : Subsystem  Commented=on
  Override  ESSOverTemp : Subsystem  Commented=on
  Override  EngOverTemp : Subsystem  Commented=on
  Override  EngTrqMismatch : Subsystem  Commented=on
  Override  LossCAN : Subsystem  Commented=on
  Override  MCUOverTemp : Subsystem  Commented=on
  Override  MotDirMismatch : Subsystem  Commented=on
  Override  MotOverTemp : Subsystem  Commented=on
  Override  MotTrqMismatch : Subsystem  Commented=on
  wires:
  MotOverTemp/1 -> Override  MotOverTemp/1(In1)
  LossCAN/1 -> Override  LossCAN/1(In1)
  time/1 -> LossCAN/1, MotTrqMismatch/1, EngTrqMismatch/1, MotOverTemp/1, MCUOverTemp/1, EngOverTemp/1, ClutchEngag/1, ESSOverTemp/1, MotDirMismatch/1
  Override  LossCAN/1(Out1) -> Goto2/1
  Override  MCUOverTemp/1(Out1) -> Goto5/1
  Override  EngTrqMismatch/1(Out1) -> Goto3/1
  Override  MotDirMismatch/1(Out1) -> Goto6/1
  MotDirMismatch/1 -> Override  MotDirMismatch/1(In1)
  Override  MotTrqMismatch/1(Out1) -> Goto1/1
  MotTrqMismatch/1 -> Mismch type1/1(In1)
  EngTrqMismatch/1 -> Mismch type/1(In1)
  Override  MotOverTemp/1(Out1) -> Goto4/1
  MCUOverTemp/1 -> Override  MCUOverTemp/1(In1)
  Override  EngOverTemp/1(Out1) -> Goto7/1
  EngOverTemp/1 -> Override  EngOverTemp/1(In1)
  Override  ESSOverTemp/1(Out1) -> Goto8/1
  ESSOverTemp/1 -> Override  ESSOverTemp/1(In1)
  Override  ClutchEngag/1(Out1) -> Goto9/1
  ClutchEngag/1 -> Override  ClutchEngag/1(In1)
  Mismch type/1(Out1) -> Override  EngTrqMismatch/1(In1)
  Mismch type1/1(Out1) -> Override  MotTrqMismatch/1(In1)

== system P2_SIL_Model_Diag/Fault Trigger Unit/Driver Interface Diagnostics setting ==
  time : Inport
  APP1_OOR : Lookup  Commented=on  InputValues=time  Table=APP1_OOR  LookUpMeth=Interpolation-Use End Values  OutDataTypeStr=int8
  APP2_OOR : Lookup  Commented=on  InputValues=time  Table=APP2_OOR  LookUpMeth=Interpolation-Use End Values  OutDataTypeStr=int8
  APP_Mismatch : Lookup  Commented=on  InputValues=time  Table=APP_Mismatch  LookUpMeth=Interpolation-Use End Values  OutDataTypeStr=int8
  BPP_Flt : Lookup  Commented=on  InputValues=time  Table=BPP_Flt  LookUpMeth=Interpolation-Use End Values  OutDataTypeStr=int8
  Goto1 : Goto  Commented=on  GotoTag=APP1_OOR_ON  TagVisibility=global
  Goto3 : Goto  Commented=on  GotoTag=BPP_Flt  TagVisibility=global
  Goto4 : Goto  Commented=on  GotoTag=KeyPos_Flt_ON  TagVisibility=global
  Goto5 : Goto  Commented=on  GotoTag=PRNDL_Flt_ON  TagVisibility=global
  Goto6 : Goto  Commented=on  GotoTag=APP2_OOR_ON  TagVisibility=global
  Goto7 : Goto  Commented=on  GotoTag=Mismatch_APP_ON  TagVisibility=global
  KeyPos_Flt : Lookup  Commented=on  InputValues=time  Table=KeyPos_Flt  LookUpMeth=Interpolation-Use End Values  OutDataTypeStr=int8
  Override  APP1_OOR : Subsystem  Commented=on
  Override  APP2_OOR : Subsystem  Commented=on
  Override  APP_Mismatch : Subsystem  Commented=on
  Override  BPP_Flt : Subsystem  Commented=on
  Override  KeyPos_Flt : Subsystem  Commented=on
  Override  PRNDL_Flt : Subsystem  Commented=on
  PRNDL_Flt : Lookup  Commented=on  InputValues=time  Table=PRNDL_Flt  LookUpMeth=Interpolation-Use End Values  OutDataTypeStr=int8
  To Workspace : ToWorkspace  Commented=on  VariableName=APP_Mismatch  SaveFormat=Timeseries  SampleTime=-1
  wires:
  PRNDL_Flt/1 -> Override  PRNDL_Flt/1(In1)
  Override  KeyPos_Flt/1(Out1) -> Goto4/1
  BPP_Flt/1 -> Override  BPP_Flt/1(In1)
  APP1_OOR/1 -> Override  APP1_OOR/1(In1)
  Override  APP1_OOR/1(Out1) -> Goto1/1
  APP2_OOR/1 -> Override  APP2_OOR/1(In1)
  Override  APP2_OOR/1(Out1) -> Goto6/1
  Override  BPP_Flt/1(Out1) -> Goto3/1
  Override  PRNDL_Flt/1(Out1) -> Goto5/1
  time/1 -> APP_Mismatch/1, APP2_OOR/1, PRNDL_Flt/1, KeyPos_Flt/1, BPP_Flt/1, APP1_OOR/1
  KeyPos_Flt/1 -> Override  KeyPos_Flt/1(In1)
  Override  APP_Mismatch/1(Out1) -> To Workspace/1, Goto7/1
  APP_Mismatch/1 -> Override  APP_Mismatch/1(In1)

== system P2_SIL_Model_Diag/Plant Actuators/Analog ==
  In1 : Inport
  APP_Fault_Insertion : Subsystem
  APP_to_APP1_Recast : Subsystem
  APP_to_APP2_Recast : Subsystem
  Bus Creator : BusCreator  Inputs=5
  Bus Creator1 : BusCreator  Inputs=2
  Bus Selector : BusSelector  OutputSignals=drv_APP_req_[%],ShiftLvrPos,KeyPos,drv_BPP_req_[%]
  Switch : Switch  Criteria=u2 > Threshold
  Out1 : Outport
  wires:
  Bus Creator/1 -> Out1/1  "Analog"
  Bus Selector/4 -> Bus Creator/5  "<drv_BPP_req_[%]>"
  Bus Selector/3 -> Bus Creator/4  "<KeyPos>"
  Bus Selector/2 -> Bus Creator/3  "<ShiftLvrPos>"
  In1/1 -> Bus Selector/1
  Bus Selector/1 -> Bus Creator/1, APP_Fault_Insertion/1(AccPos)  "<drv_APP_req_[%]>"
  APP_Fault_Insertion/1(APP1) -> APP_to_APP1_Recast/1(APP1_IN)
  APP_Fault_Insertion/2(APP2) -> APP_to_APP2_Recast/1(APP2_IN)
  APP_to_APP1_Recast/1(APP1Recast) -> Bus Creator1/1  "Driver_APP1"
  APP_to_APP2_Recast/1(APP2Recast) -> Bus Creator1/2  "Driver_APP2"
  Bus Creator1/1 -> Bus Creator/2  "APP_Out"

== system P2_SIL_Model_Diag/Plant Actuators/CAN ==
  In1 : Inport
  Bus Creator : BusCreator  Inputs=3
  EBCAN : Subsystem
  HV_CAN : Subsystem
  VEH_CAN : Subsystem
  Out1 : Outport
  wires:
  Bus Creator/1 -> Out1/1
  HV_CAN/1(Out1) -> Bus Creator/3
  EBCAN/1(Out1) -> Bus Creator/2
  VEH_CAN/1(Out1) -> Bus Creator/1
  In1/1 -> VEH_CAN/1(In1), EBCAN/1(In1), HV_CAN/1(In1)

== system P2_SIL_Model_Diag/Plant Actuators/Digital ==
  In1 : Inport
  Bus Creator : BusCreator  Inputs=3
  Bus Selector : BusSelector  OutputSignals=CS_Switch,CD_RSwitch,CS_FSwitch
  Out1 : Outport
  wires:
  Bus Creator/1 -> Out1/1  "Digital"
  Bus Selector/3 -> Bus Creator/3  "<CS_FSwitch>"
  Bus Selector/2 -> Bus Creator/2  "<CD_RSwitch>"
  Bus Selector/1 -> Bus Creator/1  "<CS_Switch>"
  In1/1 -> Bus Selector/1

== system P2_SIL_Model_Diag/Plant Sensors/Analog ==
  In1 : Inport
  Out1 : Outport
  wires:
  In1/1 -> Out1/1

== system P2_SIL_Model_Diag/Plant Sensors/CAN ==
  In1 : Inport
  Bus Creator : BusCreator  Inputs=3
  EBCAN : Subsystem
  HV_CAN : Subsystem
  VEH_CAN : Subsystem
  Out1 : Outport
  wires:
  Bus Creator/1 -> Out1/1
  HV_CAN/1(Out1) -> Bus Creator/3  "to HV_CAN"
  EBCAN/1(Out1) -> Bus Creator/2  "to EBCAN"
  VEH_CAN/1(Out1) -> Bus Creator/1  "to VEH_CAN"
  In1/1 -> VEH_CAN/1(In1), HV_CAN/1(In1), EBCAN/1(In1)

== system P2_SIL_Model_Diag/Plant Sensors/Digital ==
  In1 : Inport
  Out1 : Outport
  wires:
  In1/1 -> Out1/1

== system P2_SIL_Model_Diag/Sensors/Analog ==
  In1 : Inport
  APP Manipulation : Subsystem  AncestorBlock=lib_APP_Conversion_IN/APP_Conversion_IN
  Bus Creator : BusCreator  Inputs=5
  Bus Selector : BusSelector  OutputSignals=APP_Out.Driver_APP1,APP_Out.Driver_APP2,drv_APP_req_[%],ShiftLvrPos,KeyPos,drv_BPP_req_[%]
  Out1 : Outport
  wires:
  Bus Creator/1 -> Out1/1
  In1/1 -> Bus Selector/1
  Bus Selector/4 -> Bus Creator/3  "<ShiftLvrPos>"
  Bus Selector/5 -> Bus Creator/4  "<KeyPos>"
  Bus Selector/6 -> Bus Creator/5  "<drv_BPP_req_[%]>"
  Bus Selector/1 -> APP Manipulation/1(APP1_IN)  "<Driver_APP1>"
  Bus Selector/2 -> APP Manipulation/2(APP2_IN)  "<Driver_APP2>"
  APP Manipulation/1(APP) -> Bus Creator/2  "Com_APP"
  Bus Selector/3 -> Bus Creator/1  "<drv_APP_req_[%]>"

== system P2_SIL_Model_Diag/Sensors/CAN ==
  In1 : Inport
  Bus Creator : BusCreator  Inputs=3
  EBCAN : Subsystem
  HV_CAN : Subsystem
  VEH_CAN : Subsystem
  Out1 : Outport
  wires:
  VEH_CAN/1(Out1) -> Bus Creator/1  "fromVEH_CAN"
  Bus Creator/1 -> Out1/1  "from_CAN"
  EBCAN/1(Out1) -> Bus Creator/2  "fromEBCAN"
  HV_CAN/1(Out1) -> Bus Creator/3  "fromHV_CAN"
  In1/1 -> HV_CAN/1(In1), EBCAN/1(In1), VEH_CAN/1(In1)

== system P2_SIL_Model_Diag/Sensors/Digital ==
  In1 : Inport
  Out1 : Outport

== system P2_SIL_Model_Diag/Actuators/CAN/EBCAN ==
  In1 : Inport
  BMS_Antrieb : Subsystem
  Bus Creator : BusCreator  Inputs=2
  ECM : Subsystem
  Out1 : Outport
  wires:
  ECM/1(Out1) -> Bus Creator/1
  BMS_Antrieb/1(Out1) -> Bus Creator/2
  Bus Creator/1 -> Out1/1
  In1/1 -> BMS_Antrieb/1(In1), ECM/1(In1)

== system P2_SIL_Model_Diag/Actuators/CAN/HV_CAN ==
  In1 : Inport
  APM : Subsystem  Commented=on
  BMS_Hybrid : Subsystem
  Bus Creator : BusCreator  Inputs=4
  MCU : Subsystem
  OBC : Subsystem
  Out1 : Outport
  wires:
  BMS_Hybrid/1(Out1) -> Bus Creator/1  "to_BMS_Hybrid"
  MCU/1(Out1) -> Bus Creator/2  "to_MCU"
  OBC/1(Out1) -> Bus Creator/3  "to_OBC"
  Bus Creator/1 -> Out1/1
  APM/1(Out1) -> Bus Creator/4  "to_APM"
  In1/1 -> APM/1(In1), OBC/1(In1), MCU/1(In1), BMS_Hybrid/1(In1)

== system P2_SIL_Model_Diag/Actuators/CAN/VEH_CAN ==
  note: //*Divide the signals out of the Input by component before sending them in the TCM, EBCM etc blocks*//
  In1 : Inport
  BCM : Subsystem
  Bus Creator : BusCreator  Inputs=4
  EBCM : Subsystem
  Ground1 : Ground
  Ground2 : Ground
  ICCM : Subsystem
  TCM : Subsystem
  Out1 : Outport
  wires:
  ICCM/1(Out1) -> Bus Creator/4  "HAct_to_ICCM"
  BCM/1(Out1) -> Bus Creator/3  "HAct_to_BCM"
  EBCM/1(Out1) -> Bus Creator/2  "HAct_to_EBCM"
  TCM/1(Out1) -> Bus Creator/1  "HAct_to_TCM"
  Bus Creator/1 -> Out1/1
  In1/1 -> TCM/1(In1), BCM/1(In1)
  Ground1/1 -> EBCM/1(In1)
  Ground2/1 -> ICCM/1(In1)

== system P2_SIL_Model_Diag/Camaro Plant Model/Chassis1/Driver Interface ==
  Bus Selector1 : BusSelector  OutputSignals=KeyPos,drv_APP_req_[%],drv_BPP_req_[%],ShiftLvrPos,EVSE_Plugged
  tag scope: EVSEPlugged=global, KeyPosition=global, ShftLvrPos=global, drv_APP_percent2=global, drv_APP_percent=global, drv_BPP_percent=global
  wires:
  Bus Selector1/1 -> [KeyPosition]  "<KeyPos>"
  Bus Selector1/2 -> [drv_APP_percent], [drv_APP_percent2]  "<drv_APP_req_[%]>"
  Bus Selector1/4 -> [ShftLvrPos]  "<ShiftLvrPos>"
  [Driver_Request] -> Bus Selector1/1
  Bus Selector1/3 -> [drv_BPP_percent]  "<drv_BPP_req_[%]>"
  Bus Selector1/5 -> [EVSEPlugged]  "<EVSE_Plugged>"

== system P2_SIL_Model_Diag/Camaro Plant Model/Chassis1/Soft BCM ==
  note: This signal will go to ECM to be transmitted out
      | in the CAN message of PPEI_Vehicle_Speed_and_Distance
  note: Key Position information is collected by BCM and then sent out to HCU by BCM
      | in the CAN message of PPEI_Platforma_General_Status
  Bus Creator : BusCreator  Inputs=2
  Constant : Constant  Value=2
  Data Type Conversion1 : DataTypeConversion
  Data Type Conversion2 : DataTypeConversion
  Data Type Conversion3 : DataTypeConversion
  Data Type Conversion4 : DataTypeConversion  OutDataTypeStr=int8
  Sum : Sum  Inputs=|++
  Switch : Switch  Threshold=1
  Out1 : Outport
  tag scope: VehSpdAvgDrvn=global
  wires:
  [chas_plant_lin_spd_out] -> Data Type Conversion1/1
  Data Type Conversion1/1 -> [VehSpdAvgDrvn]
  [KeyPosition] -> Data Type Conversion2/1
  Data Type Conversion2/1 -> Switch/3, Sum/2  "SysPwrMd"
  Bus Creator/1 -> Out1/1  "BCM_CAN"
  [drv_BPP_percent] -> Data Type Conversion3/1
  Data Type Conversion3/1 -> Bus Creator/2  "BrkPdlPos"
  [KeyPos_Flt_ON] -> Switch/2
  Sum/1 -> Switch/1
  Switch/1 -> Bus Creator/1  "SysPwrMd"
  Constant/1 -> Data Type Conversion4/1
  Data Type Conversion4/1 -> Sum/1

== system P2_SIL_Model_Diag/Camaro Plant Model/Chassis1/non-zero division1 ==
  note: and finally, the expression is: (u[1] \ u[2]) * 1 = u[1] \ u[2]
  note: (u[2]!=0) is true then returns 1
  note: if u[2] != 0, then output == u[1]\u[2]:
  note: (u[2]==0) is false then returns 0, thus (u[2]+(u[2]==0)) is equal to u[2]+0=u[2]
  note: and finally, the expression is: (u[1] \ 1) * 0 = 0
  note: (u[2]!=0) is false then returns 0
  note: if u[2] == 0, then output == 0:
  note: (u[2]==0) is true then returns 1, thus (u[2]+(u[2]==0)) is equal to 0+1=1
  In1 : Inport
  In2 : Inport  Port=2
  Fcn : Fcn  Expr=u[1]/(u[2]+(u[2]==0))*(u[2]!=0)
  Mux : Mux  Inputs=2
  Out1 : Outport
  wires:
  In2/1 -> Mux/2
  Fcn/1 -> Out1/1
  In1/1 -> Mux/1
  Mux/1 -> Fcn/1

== system P2_SIL_Model_Diag/Camaro Plant Model/Chassis1/vehicle losses ==
  veh spd simu : Inport
  Road grade : Inport  Port=2
  Bus Creator : BusCreator  Inputs=2
  Drag Force Calculation : Product  Inputs=5  SaturateOnIntegerOverflow=on  InputSameDT=on  OutDataTypeStr=Inherit: Same as first input
  Grade Force Calculation : Product  Inputs=3  SaturateOnIntegerOverflow=on  InputSameDT=on  OutDataTypeStr=Inherit: Same as first input
  Product1 : Product  SaturateOnIntegerOverflow=on  InputSameDT=on  OutDataTypeStr=Inherit: Same as first input
  Sign : Signum
  Sum3 : Sum  Inputs=|++  SaturateOnIntegerOverflow=on  InputSameDT=on  OutDataTypeStr=Inherit: Same as first input
  Trigonometric Function : Trigonometry
  f1 : Constant  Value=rho
  f2 : Constant  Value=0.5
  f4 : Constant  Value=g
  mass : Constant  Value=chas.plant.init.mass.body
  mass1 : Constant  Value=chas.plant.init.area_drag
  info : Outport
  veh_force_loss_simu : Outport  Port=2
  wires:
  Bus Creator/1 -> info/1
  Sum3/1 -> veh_force_loss_simu/1  "veh_drag_and_Rx_simu"
  Grade Force Calculation/1 -> Bus Creator/1, Sum3/1  "veh_grade_force_simu"
  veh spd simu/1 -> Sign/1, Drag Force Calculation/1, Drag Force Calculation/2
  Drag Force Calculation/1 -> Product1/2, Bus Creator/2  "drag force"
  Road grade/1 -> Trigonometric Function/1
  Sign/1 -> Product1/1
  Product1/1 -> Sum3/2
  mass/1 -> Grade Force Calculation/1
  f4/1 -> Grade Force Calculation/2
  Trigonometric Function/1 -> Grade Force Calculation/3
  f1/1 -> Drag Force Calculation/4
  mass1/1 -> Drag Force Calculation/5
  f2/1 -> Drag Force Calculation/3

== system P2_SIL_Model_Diag/Camaro Plant Model/DC-DC Converter1/Subsystem2 ==
  In1 : Inport
  In2 : Inport  Port=2
  Fcn : Fcn  Expr=u[1]/(u[2]+eps)*(u[2]!=0)
  Mux : Mux  Inputs=2
  Out1 : Outport
  wires:
  In2/1 -> Mux/2
  Fcn/1 -> Out1/1
  In1/1 -> Mux/1
  Mux/1 -> Fcn/1

== system P2_SIL_Model_Diag/Camaro Plant Model/Differential/Inertia calculation ==
  inertia in : Inport
  Final Drive inertia : Constant  Value=fd.plant.init.inertia
  Sum3 : Sum  Inputs=|++  SaturateOnIntegerOverflow=on  InputSameDT=on  OutDataTypeStr=Inherit: Same as first input
  fd.plant.init.ratio : Gain  Gain=fd.plant.init.ratio  SaturateOnIntegerOverflow=on  OutDataTypeStr=Inherit: Same as input  ParamDataTypeStr=Inherit: Same as input
  "fd.plant.init.ratio " : Gain  Gain=fd.plant.init.ratio  SaturateOnIntegerOverflow=on  OutDataTypeStr=Inherit: Same as input  ParamDataTypeStr=Inherit: Same as input
  inertia out : Outport
  wires:
  inertia in/1 -> fd.plant.init.ratio/1
  "fd.plant.init.ratio "/1 -> Sum3/1
  Final Drive inertia/1 -> Sum3/2
  Sum3/1 -> inertia out/1
  fd.plant.init.ratio/1 -> "fd.plant.init.ratio "/1

== system P2_SIL_Model_Diag/Camaro Plant Model/Differential/Speed calculation ==
  spd out : Inport
  fd.plant.init.ratio : Gain  Gain=fd.plant.init.ratio  SaturateOnIntegerOverflow=on  OutDataTypeStr=Inherit: Same as input  ParamDataTypeStr=Inherit: Same as input
  spd in : Outport
  wires:
  spd out/1 -> fd.plant.init.ratio/1
  fd.plant.init.ratio/1 -> spd in/1

== system P2_SIL_Model_Diag/Camaro Plant Model/Differential/Torque calculation ==
  spd in : Inport
  trq in : Inport  Port=2
  Abs : Abs  SaturateOnIntegerOverflow=on
  Abs1 : Abs  SaturateOnIntegerOverflow=on
  Blending (state dependent) : Subsystem  mask(State dependent blending){xl=-fd.plant.init.spd_thresh, yl=-1, xc=0, yc=0, xr=fd.plant.init.spd_thresh, yr=1}
      mask prompts: xl "Left point (x):"; yl "Left point (y):"; xc "Center point (x):"; yc "Center point (y):"; xr "Right point (x):"; yr "Right point (y):"
      mask help: This block implements state dependent smoothing/blending. IMPORTANT: See help menu.
      mask Help: The output equals the product of the first input and a "hat" function defined by the three points specified in the dialog box.  The second input forms the argument to the hat function.\n\nIMPORTANT: A divide by zero error will result if first coordinates of the three points specified for the hat function are NOT distinct.
      mask Display: plot([-1 1 3 6 8], [1.5 1.5 0.5 4.0 4.0])
  Look-Up Table (2-D) : Subsystem  mask(Lookup Table (2-D)){x=fd.plant.init.trq_loss.idx1_trq, y=fd.plant.init.trq_loss.idx2_spd, t=fd.plant.init.trq_loss.map}
      mask prompts: x "Row:"; y "Column:"; t "Table:"
      mask help: Performs 2-D linear interpolation of input values using the specified input/output table. Extrapolation is performed outside the table boundaries.
      mask init:
      | [r,c]=size(t);
      | xt=reshape(x,prod(size(x)),1);
      | xi=xt(:,ones(1,c));
      | minx=min(x); maxx=max(x);
      | mint=min(min(t)); maxt=max(max(t));
      mask Display: plot(xi,t,[minx maxx],[mint mint],[minx minx],[mint maxt])
  Sum2 : Sum  Inputs=|+-  SaturateOnIntegerOverflow=on  InputSameDT=on  OutDataTypeStr=Inherit: Same as first input
  fd.plant.init.ratio : Gain  Gain=fd.plant.init.ratio  SaturateOnIntegerOverflow=on  OutDataTypeStr=Inherit: Same as input  ParamDataTypeStr=Inherit: Same as input
  trq out : Outport
  wires:
  Abs/1 -> Look-Up Table (2-D)/1(Rows)
  Abs1/1 -> Look-Up Table (2-D)/2(Cols)
  Look-Up Table (2-D)/1(Out1) -> Blending (state dependent)/1(Input)
  Blending (state dependent)/1(Output) -> Sum2/2
  trq in/1 -> Abs/1, Sum2/1
  spd in/1 -> Abs1/1, Blending (state dependent)/2(Control (state))
  Sum2/1 -> fd.plant.init.ratio/1
  fd.plant.init.ratio/1 -> trq out/1
